simulink model "Crank_and_rod_POG_mdl"  (R2019a)
settings: Solver=ode45  StartTime=0.0  StopTime=10.0  RelTol=1e-3  EnableMultiTasking=on
values from neighbouring files (symbols this model uses):
  bm = 0    [Crank_and_rod_POG_mola.m]    (also in tarefa3.m)
  bp = 0    [Crank_and_rod_POG_mola.m]    (also in tarefa3.m)
  dot_H_th_out = double(subs(dot_H_th,th))    [Crank_and_rod_POG_mola.m]    (also in tarefa3.m)
  Fp = 0    [Crank_and_rod_POG_mola.m]    (also in tarefa3.m)
  H_th_out = double(subs(H_th,th))    [Crank_and_rod_POG_mola.m]    (also in tarefa3.m)
  Jm = 0.0013    [Crank_and_rod_POG_mola.m]    (also in tarefa3.m)
  k = 10    [Crank_and_rod_POG_mola.m]    (also in SS.m = 3; TF.m = 3; tarefa3.m)
  mp = 0.8    [Crank_and_rod_POG_mola.m]    (also in tarefa3.m)
  Tc = Tfin/4000    (= 0.0025)    [Crank_and_rod_POG_mola.m]    (also in tarefa3.m)
  Th_in = th    [Crank_and_rod_POG_mola.m]    (also in tarefa3.m)
  Thm_0 = 0    [Crank_and_rod_POG_mola.m]    (also in tarefa3.m)
  Tm = 0    [Crank_and_rod_POG_mola.m]    (also in tarefa3.m)
  Wm_0 = 20.944    [Crank_and_rod_POG_mola.m]    (also in tarefa3.m)
settings Model: Creator=roberto  LastModifiedBy=rubiarg
settings DataIOCC: LimitDataPoints=on  SaveFormat=Array  SignalLoggingSaveFormat=ModelDataLogs  ReturnWorkspaceOutputs=off
settings OptimizationCC: ExpressionDepthLimit=2147483647  InitFltsAndDblsToZero=on  LifeSpan=inf
settings DebuggingCC: SaveWithParameterizedLinksMsg=none  UnderspecifiedInitializationDetection=Classic  MergeDetectMultiDrivingBlocksExec=none  SignalResolutionControl=TryResolveAllWithWarning  SolverPrmCheckMsg=warning  MultiTaskDSMMsg=warning  MultiTaskCondExecSysMsg=none  FcnCallInpInsideContextMsg=warning  StateNameClashWarn=warning  SFUnexpectedBacktrackingDiag=warning  SFNoUnconditionalDefaultTransitionDiag=warning  SFExecutionAtInitializationDiag=none  ArithmeticOperatorsInVariantConditions=warning
settings HardwareCC: ProdBitPerPointer=32  ProdBitPerSizeT=32  ProdBitPerPtrDiffT=32  ProdLargestAtomicFloat=None  ProdIntDivRoundTo=Undefined  ProdEndianess=Unspecified  ProdWordSize=32  ProdHWDeviceType=32-bit Generic
settings ModelReferenceCC: PropagateSignalLabelsOutOfModel=off
settings SFSimCC: SimUseLocalCustomCode=off
settings RTWCC: RTWUseLocalCustomCode=off
settings CodeAppCC: StateflowObjectComments=on
settings GRTTargetCC: TargetFcnLib=ansi_tfl_tmw.mat  TargetLangStandard=C89/C90 (ANSI)  GeneratePreprocessorConditionals=Disable all  CombineOutputUpdateFcns=off  GRTInterface=on
settings ConfigComp: CovMetricSettings=dw  CovHtmlReporting=on  CovSaveCumulativeToWorkspaceVar=on  CovSaveSingleToWorkspaceVar=on  CovExternalEMLEnable=off

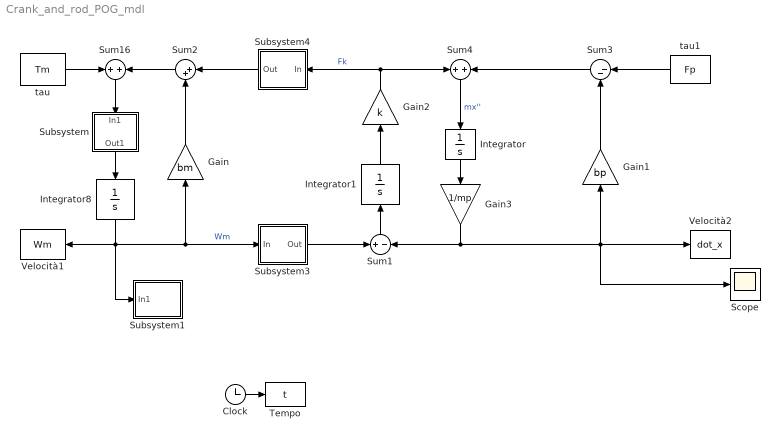
== system Crank_and_rod_POG_mdl ==
  Clock : Clock
  Gain : Gain  Gain=bm
  Gain1 : Gain  Gain=bp
  Gain2 : Gain  Gain=k
  Gain3 : Gain  Gain=1/mp
  Integrator : Integrator
  Integrator1 : Integrator  LowerSaturationLimit=0
  Integrator8 : Integrator  InitialCondition=Wm_0  LowerSaturationLimit=0
  Scope : Scope
  Subsystem : Subsystem
      mask Display: disp('1/J(th)')
  Subsystem1 : Subsystem
      mask Display: disp('H(th),  \n dH(th)/dt')
  Subsystem3 : Subsystem
      mask Display: disp('H(th)')
  Subsystem4 : Subsystem
      mask Display: disp('H(th)')
  Sum1 : Sum  Inputs=+|-
  Sum16 : Sum  Inputs=+|+
  Sum2 : Sum  Inputs=|++
  Sum3 : Sum  Inputs=|--
  Sum4 : Sum  Inputs=+|+
  Tempo : ToWorkspace  VariableName=t  SampleTime=Tc
  Velocità1 : ToWorkspace  VariableName=Wm  SampleTime=Tc
  Velocità2 : ToWorkspace  VariableName=dot_x  SampleTime=Tc
  tau : Constant  Value=Tm
  tau1 : Constant  Value=Fp
  wires:
  Clock/1 -> Tempo/1
  Integrator8/1 -> Velocità1/1, Subsystem3/1(In), Gain/1, Subsystem1/1(In1)  "Wm"
  Sum2/1 -> Sum16/2
  tau/1 -> Sum16/1
  Gain/1 -> Sum2/2
  Subsystem4/1(Out) -> Sum2/1
  Gain1/1 -> Sum3/2
  tau1/1 -> Sum3/1
  Sum16/1 -> Subsystem/1(In1)
  Subsystem/1(Out1) -> Integrator8/1
  Integrator1/1 -> Gain2/1
  Subsystem3/1(Out) -> Sum1/1
  Sum1/1 -> Integrator1/1
  Integrator/1 -> Gain3/1
  Gain3/1 -> Sum1/2, Scope/1, Velocità2/1, Gain1/1
  Sum4/1 -> Integrator/1  "mx''"
  Sum3/1 -> Sum4/2
  Gain2/1 -> Sum4/1, Subsystem4/1(In)  "Fk"

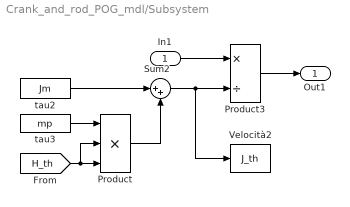
== system Crank_and_rod_POG_mdl/Subsystem ==
  In1 : Inport
  Product : Product  Inputs=3  RndMeth=Zero
  Product3 : Product  Inputs=*/  RndMeth=Zero
  Sum2 : Sum  Inputs=|++
  Velocità2 : ToWorkspace  VariableName=J_th  SampleTime=Tc
  tau2 : Constant  Value=Jm
  tau3 : Constant  Value=mp
  Out1 : Outport
  wires:
  tau3/1 -> Product/1
  [H_th] -> Product/2, Product/3
  tau2/1 -> Sum2/1
  Product/1 -> Sum2/2
  Sum2/1 -> Product3/2, Velocità2/1
  In1/1 -> Product3/1
  Product3/1 -> Out1/1

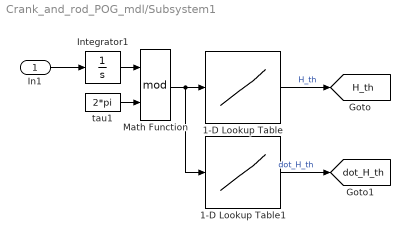
== system Crank_and_rod_POG_mdl/Subsystem1 ==
  In1 : Inport
  1-D Lookup Table : Lookup_n-D  NumberOfTableDimensions=1  BreakpointsForDimension1=Th_in  Table=H_th_out  RndMeth=Simplest  InputSameDT=on
  1-D Lookup Table1 : Lookup_n-D  NumberOfTableDimensions=1  BreakpointsForDimension1=Th_in  Table=dot_H_th_out  RndMeth=Simplest  InputSameDT=on
  Integrator1 : Integrator  InitialCondition=Thm_0  LowerSaturationLimit=0
  Math Function : Math  Operator=mod  SaturateOnIntegerOverflow=on
  tau1 : Constant  Value=2*pi
  tag scope: H_th=global, dot_H_th=global
  wires:
  Integrator1/1 -> Math Function/1
  tau1/1 -> Math Function/2
  Math Function/1 -> 1-D Lookup Table/1, 1-D Lookup Table1/1
  1-D Lookup Table/1 -> [H_th]  "H_th"
  1-D Lookup Table1/1 -> [dot_H_th]  "dot_H_th"
  In1/1 -> Integrator1/1

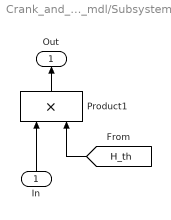
== system Crank_and_rod_POG_mdl/Subsystem3 ==
  In : Inport
  Product1 : Product  RndMeth=Zero
  Out : Outport
  wires:
  Product1/1 -> Out/1
  In/1 -> Product1/1
  [H_th] -> Product1/2

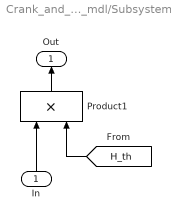
== system Crank_and_rod_POG_mdl/Subsystem4 ==
  In : Inport
  Product1 : Product  RndMeth=Zero
  Out : Outport
  wires:
  [H_th] -> Product1/2
  In/1 -> Product1/1
  Product1/1 -> Out/1
